simulink model "simularesistdiscretcuero"  (Simulink 7.2)
settings: Solver=ode45  StartTime=0.0  StopTime=10.0  RelTol=1e-3
settings Model: Creator=student  LastModifiedBy=student

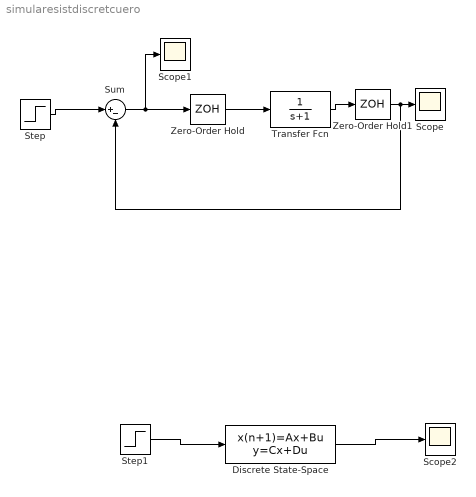
== system simularesistdiscretcuero ==
  Discrete State-Space : DiscreteStateSpace  A=[0 -0.25;1 1]  B=[1;1]  C=[0 1]  D=0  X0=[1;1]  SampleTime=0.2
  Scope : Scope
  Scope1 : Scope
  Scope2 : Scope
      settings: SaveName=ScopeData2
  Step : Step  SampleTime=0.2
  Step1 : Step  Time=0  SampleTime=0.2
  Sum : Sum  Inputs=|+-  OutDataType=sfix(16)  OutScaling=2^0
  Transfer Fcn : TransferFcn  Denominator=[1 1]
  Zero-Order Hold : ZeroOrderHold  SampleTime=0.2
  Zero-Order Hold1 : ZeroOrderHold  SampleTime=0.2
  wires:
  Step/1 -> Sum/1
  Sum/1 -> Zero-Order Hold/1, Scope1/1
  Zero-Order Hold/1 -> Transfer Fcn/1
  Transfer Fcn/1 -> Zero-Order Hold1/1
  Zero-Order Hold1/1 -> Scope/1, Sum/2
  Step1/1 -> Discrete State-Space/1
  Discrete State-Space/1 -> Scope2/1
